simulink subsystem "Linear_Motor"  (R2022b)
settings: Solver=VariableStepAuto  StartTime=0.0  StopTime=10.0  RelTol=1e-3
model mask{motor_model=0, initial_conditions=zeros(3,1)}
  mask prompts: motor_model "Motor Parameters struct:"; initial_conditions "Motor Initial Conditions:"
undefined symbols (not defined in the file): approximate, enable_Tc, enable_Tsb, lambda, tau_c, tau_sb, w_sb
settings Model: Creator=gotta  LastModifiedBy=gotta

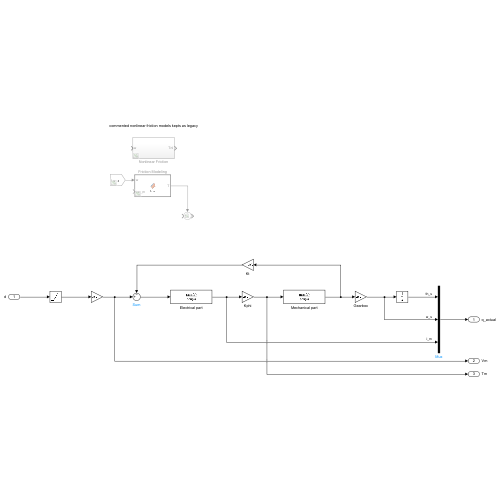
[thumbnail: Simulink's stored preview of the top-level diagram]
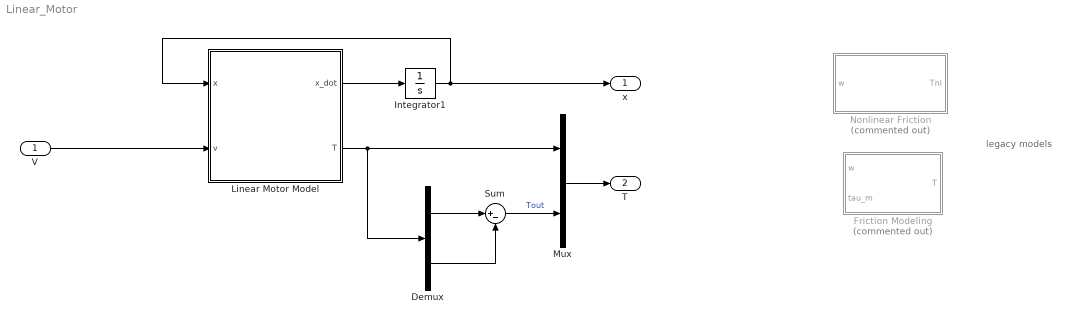
== system Linear_Motor ==
  note: legacy models
  V : Inport
  Demux : Demux  Outputs=2
  Friction Modeling : MATLAB Function  Commented=on  TreatAsAtomicUnit=on
  Integrator1 : Integrator  InitialCondition=initial_conditions
  Linear Motor Model : MATLAB Function  TreatAsAtomicUnit=on
  Mux : Mux  Inputs=2
  Nonlinear Friction : Subsystem  Commented=on
  Sum : Sum  Inputs=|+-
  x : Outport
  T : Outport  Port=2
  wires:
  Sum/1 -> Mux/2  "Tout"
  Demux/2 -> Sum/2
  Mux/1 -> T/1
  Demux/1 -> Sum/1
  Linear Motor Model/2(T) -> Mux/1, Demux/1
  Integrator1/1 -> Linear Motor Model/1(x), x/1
  Linear Motor Model/1(x_dot) -> Integrator1/1
  V/1 -> Linear Motor Model/2(v)

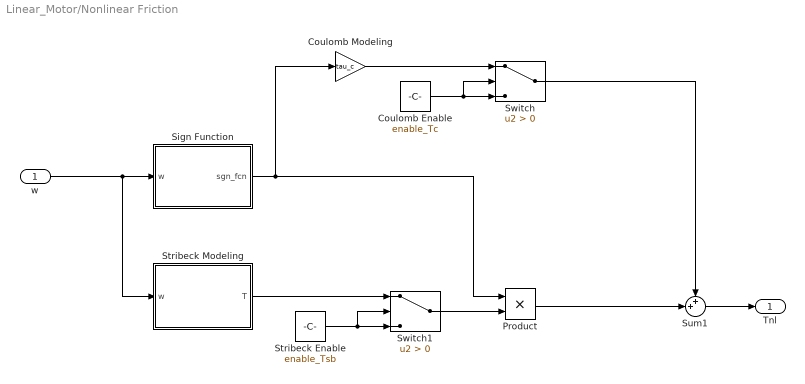
== system Linear_Motor/Nonlinear Friction ==
  w : Inport
  Coulomb Enable : Constant  Value=enable_Tc
  Coulomb Modeling : Gain  Gain=tau_c
  Product : Product
  Sign Function : MATLAB Function  TreatAsAtomicUnit=on
  Stribeck Enable : Constant  Value=enable_Tsb
  Stribeck Modeling : MATLAB Function  TreatAsAtomicUnit=on
  Sum1 : Sum  Inputs=++|
  Switch : Switch  Criteria=u2 > Threshold  SaturateOnIntegerOverflow=off  InputSameDT=off
  Switch1 : Switch  Criteria=u2 > Threshold  SaturateOnIntegerOverflow=off  InputSameDT=off
  Tnl : Outport
  wires:
  w/1 -> Stribeck Modeling/1(w), Sign Function/1(w)
  Stribeck Modeling/1(T) -> Switch1/1
  Sum1/1 -> Tnl/1
  Switch/1 -> Sum1/1
  Coulomb Modeling/1 -> Switch/1
  Coulomb Enable/1 -> Switch/2, Switch/3
  Stribeck Enable/1 -> Switch1/2, Switch1/3
  Switch1/1 -> Product/2
  Sign Function/1(sgn_fcn) -> Coulomb Modeling/1, Product/1
  Product/1 -> Sum1/2

== matlab function Linear_Motor/Friction Modeling ==
  data: w input; tau_m input; T output; tau_sb parameter; w_sb parameter; tau_c parameter; enable_Tc parameter; enable_Tsb parameter
function T = fcn(w, tau_m, tau_sb, w_sb, tau_c, enable_Tc, enable_Tsb)

T = 0; % linear model case

if (enable_Tc || enable_Tsb) 
    if abs(w) <= w_sb && abs(tau_m) <= tau_sb
        T = tau_m;
    else
        Tc = tau_c*sign(w)*enable_Tc;
        Tsb = (tau_sb - tau_c)*exp(-(w/w_sb)^2)*sign(w)*enable_Tsb;
        T = Tc + Tsb;
    end
end

== matlab function Linear_Motor/Linear Motor Model ==
  data: x input; v input; x_dot output; T output; motor_model parameter
function [x_dot, T] = motor(x, v, motor_model)

[x_dot, T] = motor_linear(x, v, motor_model);

== matlab function Linear_Motor/Nonlinear Friction/Sign Function ==
  data: w input; sgn_fcn output; approximate parameter; lambda parameter
function sgn_fcn = fcn(w, approximate, lambda)

% Sign function approximator
tan_sign = 2/(1+exp(-lambda*w)) - 1;

% Sign function selection
sgn_fcn = sign(w);
if approximate
    sgn_fcn = tan_sign;
end

== matlab function Linear_Motor/Nonlinear Friction/Stribeck Modeling ==
  data: w input; T output; tau_c parameter; tau_sb parameter; w_sb parameter
function T = fcn(w, tau_c, tau_sb, w_sb)


T = (tau_sb - tau_c)*exp(-(w / w_sb)^2);
